simulink model "sim_4_solver"  (R2022b)
settings: Solver=VariableStepAuto  StartTime=0.0  StopTime=10.0  RelTol=1e-3
undefined symbols (not defined in the file or in its folder): alpha
settings Model: Creator=user  LastModifiedBy=user

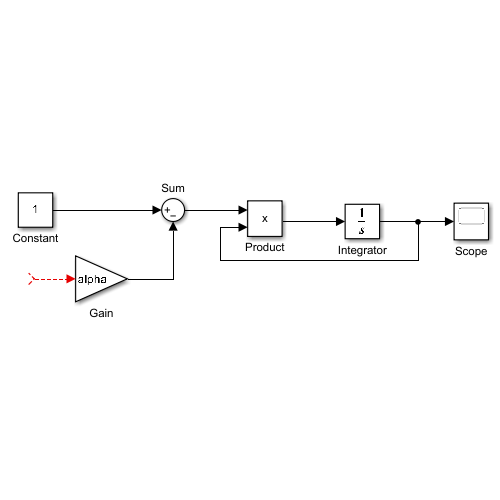
[thumbnail: Simulink's stored preview of the top-level diagram]
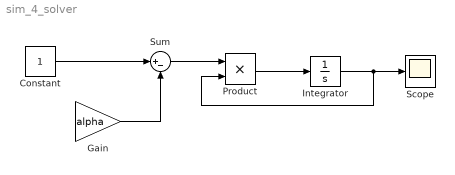
== system sim_4_solver ==
  Constant : Constant
  Gain : Gain  Gain=alpha
  Integrator : Integrator
  Product : Product
  Scope : Scope
  Sum : Sum  Inputs=|+-
  wires:
  Constant/1 -> Sum/1
  Gain/1 -> Sum/2
  ? -> Gain/1
  Sum/1 -> Product/1
  Product/1 -> Integrator/1
  Integrator/1 -> Product/2, Scope/1
